simulink model "slcrlobv"  (R2022a)
settings: Solver=FixedStepAuto  StartTime=0.0  StopTime=20  FixedStep=0.001  RelTol=1e-3
settings Model: Creator=aa211  LastModifiedBy=aa211

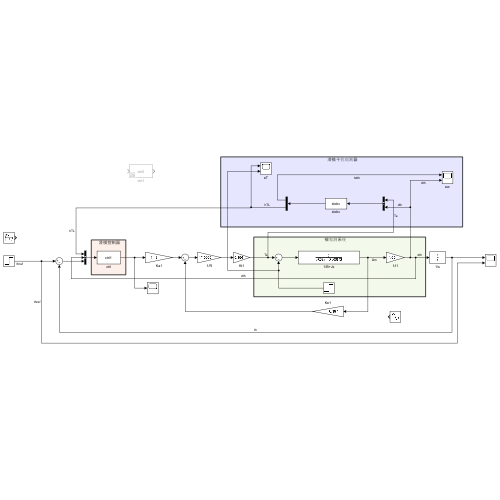
[thumbnail: Simulink's stored preview of the top-level diagram]
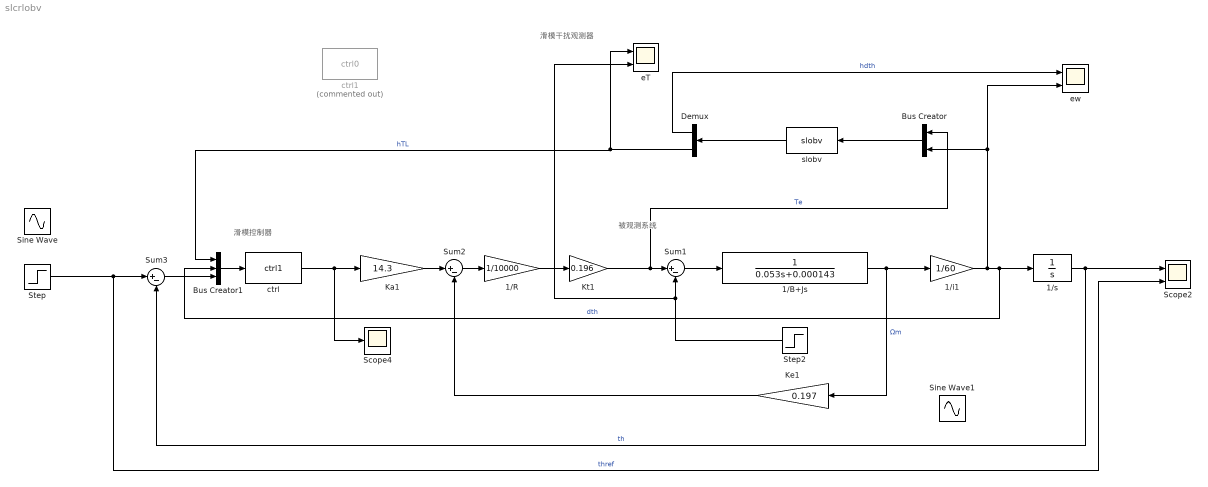
== system slcrlobv ==
  note: 被观测系统
  note: 滑模控制器
  note: 滑模干扰观测器
  1/B+Js : TransferFcn  Denominator=[0.053 0.000143]
  1/R : Gain  Gain=1/10000
  1/i1 : Gain  Gain=1/60
  1/s : TransferFcn  Denominator=[1 0]
  Bus Creator : BusCreator  Inputs=2
  Bus Creator1 : BusCreator  Inputs=3
  Demux : Demux  Outputs=2
  Ka1 : Gain  Gain=14.3
  Ke1 : Gain  Gain=0.197
  Kt1 : Gain  Gain=0.196
  Scope2 : Scope  NumInputPorts=2
  Scope4 : Scope
  Sine Wave : Sin  Amplitude=30  Frequency=1.05  SampleTime=0
  Sine Wave1 : Sin  Amplitude=5500  Frequency=5  SampleTime=0
  Step : Step  Time=0  After=30  SampleTime=0
  Step2 : Step  Time=10  After=550  SampleTime=0
  Sum1 : Sum  Inputs=|+-
  Sum2 : Sum  Inputs=|+-
  Sum3 : Sum  Inputs=|+-
  ctrl : S-Function  FunctionName=ctrl1  Parameters=pa  SFunctionDeploymentMode=off  EnableBusSupport=off
  ctrl1 : S-Function  Commented=on  FunctionName=ctrl0  Parameters=pa  SFunctionDeploymentMode=off  EnableBusSupport=off
  eT : Scope  NumInputPorts=2
  ew : Scope  NumInputPorts=2
  slobv : S-Function  FunctionName=slobv  Parameters=pa  SFunctionDeploymentMode=off  EnableBusSupport=off
  wires:
  1/s/1 -> Scope2/1, Sum3/2  "th"
  Step/1 -> Scope2/2, Sum3/1  "thref"
  ctrl/1 -> Ka1/1, Scope4/1
  Sum3/1 -> Bus Creator1/3
  Bus Creator1/1 -> ctrl/1
  Demux/1 -> ew/1  "hdth"
  1/B+Js/1 -> Ke1/1, 1/i1/1  "Ωm"
  Demux/2 -> Bus Creator1/1, eT/1  "hTL"
  Sum1/1 -> 1/B+Js/1
  Kt1/1 -> Bus Creator/1, Sum1/1  "Te"
  Ka1/1 -> Sum2/1
  1/i1/1 -> Bus Creator1/2, 1/s/1, ew/2, Bus Creator/2  "dth"
  Ke1/1 -> Sum2/2
  Step2/1 -> eT/2, Sum1/2
  Sum2/1 -> 1/R/1
  slobv/1 -> Demux/1
  Bus Creator/1 -> slobv/1
  1/R/1 -> Kt1/1
